simulink model "ex03"  (R2015b)
settings: Solver=VariableStepAuto  StartTime=0.0  StopTime=10.0  RelTol=1e-3
settings Model: Creator=Tom  LastModifiedBy=Tom

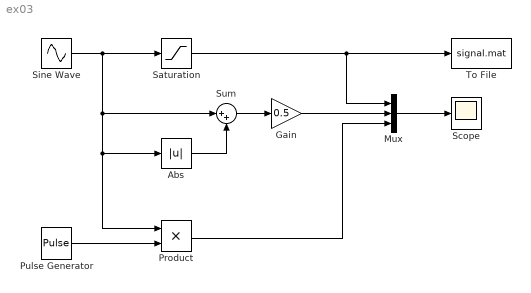
== system ex03 ==
  Abs : Abs
  Gain : Gain  Gain=0.5
  Mux : Mux  Inputs=3
  Product : Product
  Pulse Generator : DiscretePulseGenerator  PulseType=Time based  Period=2*pi  PulseWidth=50
  Saturation : Saturate  UpperLimit=Inf  LowerLimit=0
  Scope : Scope
  Sine Wave : Sin  SampleTime=0
  Sum : Sum  Inputs=|++
  To File : ToFile  Filename=signal.mat  MatrixName=signal  SaveFormat=Timeseries
  wires:
  Mux/1 -> Scope/1
  Sine Wave/1 -> Abs/1, Product/1, Sum/1, Saturation/1
  Abs/1 -> Sum/2
  Sum/1 -> Gain/1
  Pulse Generator/1 -> Product/2
  Saturation/1 -> To File/1, Mux/1
  Gain/1 -> Mux/2
  Product/1 -> Mux/3
